simulink model "ex4_planar_robot_ct_gravity_simulation"  (R2016a)
settings: Solver=FixedStepAuto  StartTime=0.0  StopTime=10  FixedStep=0.001  RelTol=1e-3
values from neighbouring files (symbols this model uses):
  a1 = u_gen(15)    [classical_joint_planar_robot_simulink.m]    (also in ct_gravit_planar_robot_simulink.m = u_gen(13); ct_pid_planar_robot_simulink.m; ct_planar_robot_simulink.m = u_gen(13); ex_planar_robot_2dof.m = 1)
  a2 = u_gen(16)    [classical_joint_planar_robot_simulink.m]    (also in ct_gravit_planar_robot_simulink.m = u_gen(14); ct_pid_planar_robot_simulink.m; ct_planar_robot_simulink.m = u_gen(14); ex_planar_robot_2dof.m = 1)
  b1 = u_gen(15)    [ct_gravit_planar_robot_simulink.m]    (also in ex_planar_robot_2dof.m = 0)
  b2 = u_gen(16)    [ct_gravit_planar_robot_simulink.m]    (also in ex_planar_robot_2dof.m = 0)
  g = u_gen(17)    [classical_joint_planar_robot_simulink.m]    (also in ct_gravit_planar_robot_simulink.m; ct_pid_planar_robot_simulink.m; ct_planar_robot_simulink.m = u_gen(15); ex_planar_robot_2dof.m = 9.81)
  m1 = u_gen(11)    [ac_controller_simulink.m]    (also in classical_joint_planar_robot_simulink.m = u_gen(13); ct_gravit_planar_robot_simulink.m; ct_pid_planar_robot_simulink.m = u_gen(13); ct_planar_robot_simulink.m)
  m2 = u_gen(12)    [ac_controller_simulink.m]    (also in classical_joint_planar_robot_simulink.m = u_gen(14); ct_gravit_planar_robot_simulink.m; ct_pid_planar_robot_simulink.m = u_gen(14); ct_planar_robot_simulink.m)
settings Model: Creator=sevimeda  LastModifiedBy=sevimeda

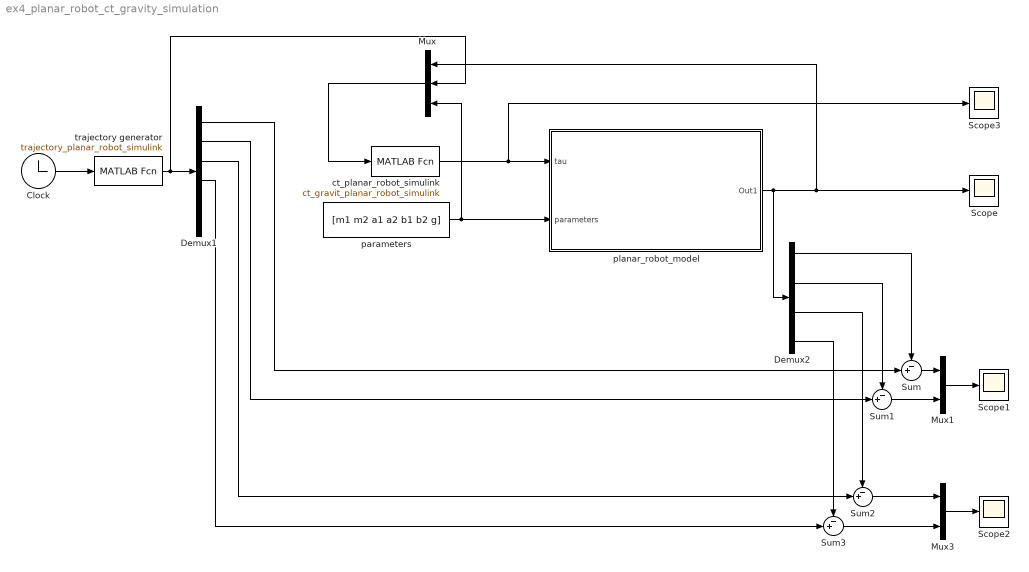
== system ex4_planar_robot_ct_gravity_simulation ==
  Clock : Clock
  Demux1 : Demux  Outputs=6
  Demux2 : Demux
  Mux : Mux  Inputs=3
  Mux1 : Mux  Inputs=2
  Mux3 : Mux  Inputs=2
  Scope{,1..3} (4 alike) : Scope
  Sum{,1..3} (4 alike) : Sum  Inputs=-+|
  ct_planar_robot_simulink : MATLABFcn  MATLABFcn=ct_gravit_planar_robot_simulink
  parameters : Constant  Value=[m1 m2 a1 a2 b1 b2 g]
  planar_robot_model : Subsystem
  trajectory generator : MATLABFcn  MATLABFcn=trajectory_planar_robot_simulink
  wires:
  Clock/1 -> trajectory generator/1
  trajectory generator/1 -> Demux1/1, Mux/2
  Mux/1 -> ct_planar_robot_simulink/1
  ct_planar_robot_simulink/1 -> Scope3/1, planar_robot_model/1(tau)
  parameters/1 -> planar_robot_model/2(parameters), Mux/3
  planar_robot_model/1(Out1) -> Mux/1, Scope/1, Demux2/1
  Demux1/1 -> Sum/2
  Demux2/1 -> Sum/1
  Demux2/2 -> Sum1/1
  Demux1/2 -> Sum1/2
  Sum2/1 -> Mux3/1
  Sum3/1 -> Mux3/2
  Demux2/3 -> Sum2/1
  Demux2/4 -> Sum3/1
  Demux1/3 -> Sum2/2
  Demux1/4 -> Sum3/2
  Mux3/1 -> Scope2/1
  Sum/1 -> Mux1/1
  Sum1/1 -> Mux1/2
  Mux1/1 -> Scope1/1

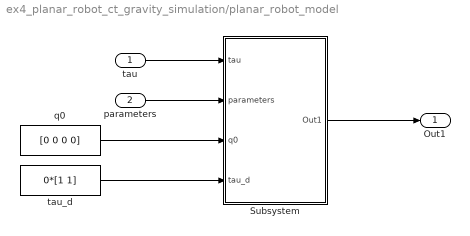
== system ex4_planar_robot_ct_gravity_simulation/planar_robot_model ==
  tau : Inport
  parameters : Inport  Port=2
  Subsystem : Subsystem
  q0 : Constant  Value=[0 0 0 0]
  tau_d : Constant  Value=0*[1 1]
  Out1 : Outport
  wires:
  Subsystem/1(Out1) -> Out1/1
  q0/1 -> Subsystem/3(q0)
  tau_d/1 -> Subsystem/4(tau_d)
  tau/1 -> Subsystem/1(tau)
  parameters/1 -> Subsystem/2(parameters)

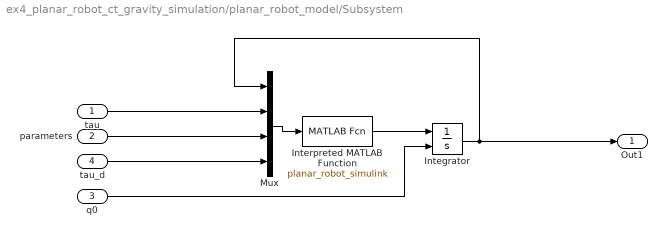
== system ex4_planar_robot_ct_gravity_simulation/planar_robot_model/Subsystem ==
  tau : Inport
  parameters : Inport  Port=2
  q0 : Inport  Port=3
  tau_d : Inport  Port=4
  Integrator : Integrator  InitialConditionSource=external
  Interpreted MATLAB Function : MATLABFcn  MATLABFcn=planar_robot_simulink  OutputDimensions=4
  Mux : Mux
  Out1 : Outport
  wires:
  Interpreted MATLAB Function/1 -> Integrator/1
  q0/1 -> Integrator/2
  Mux/1 -> Interpreted MATLAB Function/1
  Integrator/1 -> Out1/1, Mux/1
  tau/1 -> Mux/2
  parameters/1 -> Mux/3
  tau_d/1 -> Mux/4
